simulink model "BT_da_train_cach2"  (R2017b)
(part 3 of 4)

  "IW{1,1}(98,:)'"/1 -> dotprod98/1
  dotprod98/1 -> Mux/98
  "IW{1,1}(99,:)'"/1 -> dotprod99/1
  dotprod99/1 -> Mux/99
  "IW{1,1}(100,:)'"/1 -> dotprod100/1
  dotprod100/1 -> Mux/100
  "IW{1,1}(101,:)'"/1 -> dotprod101/1
  dotprod101/1 -> Mux/101
  "IW{1,1}(102,:)'"/1 -> dotprod102/1
  dotprod102/1 -> Mux/102
  "IW{1,1}(103,:)'"/1 -> dotprod103/1
  dotprod103/1 -> Mux/103
  "IW{1,1}(104,:)'"/1 -> dotprod104/1
  dotprod104/1 -> Mux/104
  "IW{1,1}(105,:)'"/1 -> dotprod105/1
  dotprod105/1 -> Mux/105
  "IW{1,1}(106,:)'"/1 -> dotprod106/1
  dotprod106/1 -> Mux/106
  "IW{1,1}(107,:)'"/1 -> dotprod107/1
  dotprod107/1 -> Mux/107
  "IW{1,1}(108,:)'"/1 -> dotprod108/1
  dotprod108/1 -> Mux/108
  "IW{1,1}(109,:)'"/1 -> dotprod109/1
  dotprod109/1 -> Mux/109
  "IW{1,1}(110,:)'"/1 -> dotprod110/1
  dotprod110/1 -> Mux/110
  "IW{1,1}(111,:)'"/1 -> dotprod111/1
  dotprod111/1 -> Mux/111
  "IW{1,1}(112,:)'"/1 -> dotprod112/1
  dotprod112/1 -> Mux/112
  "IW{1,1}(113,:)'"/1 -> dotprod113/1
  dotprod113/1 -> Mux/113
  "IW{1,1}(114,:)'"/1 -> dotprod114/1
  dotprod114/1 -> Mux/114
  "IW{1,1}(115,:)'"/1 -> dotprod115/1
  dotprod115/1 -> Mux/115
  "IW{1,1}(116,:)'"/1 -> dotprod116/1
  dotprod116/1 -> Mux/116
  "IW{1,1}(117,:)'"/1 -> dotprod117/1
  dotprod117/1 -> Mux/117
  "IW{1,1}(118,:)'"/1 -> dotprod118/1
  dotprod118/1 -> Mux/118
  "IW{1,1}(119,:)'"/1 -> dotprod119/1
  dotprod119/1 -> Mux/119
  "IW{1,1}(120,:)'"/1 -> dotprod120/1
  dotprod120/1 -> Mux/120
  "IW{1,1}(121,:)'"/1 -> dotprod121/1
  dotprod121/1 -> Mux/121
  "IW{1,1}(122,:)'"/1 -> dotprod122/1
  dotprod122/1 -> Mux/122
  "IW{1,1}(123,:)'"/1 -> dotprod123/1
  dotprod123/1 -> Mux/123
  "IW{1,1}(124,:)'"/1 -> dotprod124/1
  dotprod124/1 -> Mux/124
  "IW{1,1}(125,:)'"/1 -> dotprod125/1
  dotprod125/1 -> Mux/125
  "IW{1,1}(126,:)'"/1 -> dotprod126/1
  dotprod126/1 -> Mux/126
  "IW{1,1}(127,:)'"/1 -> dotprod127/1
  dotprod127/1 -> Mux/127
  "IW{1,1}(128,:)'"/1 -> dotprod128/1
  dotprod128/1 -> Mux/128
  "IW{1,1}(129,:)'"/1 -> dotprod129/1
  dotprod129/1 -> Mux/129
  "IW{1,1}(130,:)'"/1 -> dotprod130/1
  dotprod130/1 -> Mux/130
  "IW{1,1}(131,:)'"/1 -> dotprod131/1
  dotprod131/1 -> Mux/131
  "IW{1,1}(132,:)'"/1 -> dotprod132/1
  dotprod132/1 -> Mux/132
  "IW{1,1}(133,:)'"/1 -> dotprod133/1
  dotprod133/1 -> Mux/133
  "IW{1,1}(134,:)'"/1 -> dotprod134/1
  dotprod134/1 -> Mux/134
  "IW{1,1}(135,:)'"/1 -> dotprod135/1
  dotprod135/1 -> Mux/135
  "IW{1,1}(136,:)'"/1 -> dotprod136/1
  dotprod136/1 -> Mux/136
  "IW{1,1}(137,:)'"/1 -> dotprod137/1
  dotprod137/1 -> Mux/137
  "IW{1,1}(138,:)'"/1 -> dotprod138/1
  dotprod138/1 -> Mux/138
  "IW{1,1}(139,:)'"/1 -> dotprod139/1
  dotprod139/1 -> Mux/139
  "IW{1,1}(140,:)'"/1 -> dotprod140/1
  dotprod140/1 -> Mux/140
  "IW{1,1}(141,:)'"/1 -> dotprod141/1
  dotprod141/1 -> Mux/141
  "IW{1,1}(142,:)'"/1 -> dotprod142/1
  dotprod142/1 -> Mux/142
  "IW{1,1}(143,:)'"/1 -> dotprod143/1
  dotprod143/1 -> Mux/143
  "IW{1,1}(144,:)'"/1 -> dotprod144/1
  dotprod144/1 -> Mux/144
  "IW{1,1}(145,:)'"/1 -> dotprod145/1
  dotprod145/1 -> Mux/145
  "IW{1,1}(146,:)'"/1 -> dotprod146/1
  dotprod146/1 -> Mux/146
  "IW{1,1}(147,:)'"/1 -> dotprod147/1
  dotprod147/1 -> Mux/147
  "IW{1,1}(148,:)'"/1 -> dotprod148/1
  dotprod148/1 -> Mux/148
  "IW{1,1}(149,:)'"/1 -> dotprod149/1
  dotprod149/1 -> Mux/149
  "IW{1,1}(150,:)'"/1 -> dotprod150/1
  dotprod150/1 -> Mux/150
  "IW{1,1}(151,:)'"/1 -> dotprod151/1
  dotprod151/1 -> Mux/151
  "IW{1,1}(152,:)'"/1 -> dotprod152/1
  dotprod152/1 -> Mux/152
  "IW{1,1}(153,:)'"/1 -> dotprod153/1
  dotprod153/1 -> Mux/153
  "IW{1,1}(154,:)'"/1 -> dotprod154/1
  dotprod154/1 -> Mux/154
  "IW{1,1}(155,:)'"/1 -> dotprod155/1
  dotprod155/1 -> Mux/155
  "IW{1,1}(156,:)'"/1 -> dotprod156/1
  dotprod156/1 -> Mux/156
  "IW{1,1}(157,:)'"/1 -> dotprod157/1
  dotprod157/1 -> Mux/157
  "IW{1,1}(158,:)'"/1 -> dotprod158/1
  dotprod158/1 -> Mux/158
  "IW{1,1}(159,:)'"/1 -> dotprod159/1
  dotprod159/1 -> Mux/159
  "IW{1,1}(160,:)'"/1 -> dotprod160/1
  dotprod160/1 -> Mux/160
  "IW{1,1}(161,:)'"/1 -> dotprod161/1
  dotprod161/1 -> Mux/161
  "IW{1,1}(162,:)'"/1 -> dotprod162/1
  dotprod162/1 -> Mux/162
  "IW{1,1}(163,:)'"/1 -> dotprod163/1
  dotprod163/1 -> Mux/163
  "IW{1,1}(164,:)'"/1 -> dotprod164/1
  dotprod164/1 -> Mux/164
  "IW{1,1}(165,:)'"/1 -> dotprod165/1
  dotprod165/1 -> Mux/165
  "IW{1,1}(166,:)'"/1 -> dotprod166/1
  dotprod166/1 -> Mux/166
  "IW{1,1}(167,:)'"/1 -> dotprod167/1
  dotprod167/1 -> Mux/167
  "IW{1,1}(168,:)'"/1 -> dotprod168/1
  dotprod168/1 -> Mux/168
  "IW{1,1}(169,:)'"/1 -> dotprod169/1
  dotprod169/1 -> Mux/169
  "IW{1,1}(170,:)'"/1 -> dotprod170/1
  dotprod170/1 -> Mux/170
  "IW{1,1}(171,:)'"/1 -> dotprod171/1
  dotprod171/1 -> Mux/171
  "IW{1,1}(172,:)'"/1 -> dotprod172/1
  dotprod172/1 -> Mux/172
  "IW{1,1}(173,:)'"/1 -> dotprod173/1
  dotprod173/1 -> Mux/173
  "IW{1,1}(174,:)'"/1 -> dotprod174/1
  dotprod174/1 -> Mux/174
  "IW{1,1}(175,:)'"/1 -> dotprod175/1
  dotprod175/1 -> Mux/175
  "IW{1,1}(176,:)'"/1 -> dotprod176/1
  dotprod176/1 -> Mux/176
  "IW{1,1}(177,:)'"/1 -> dotprod177/1
  dotprod177/1 -> Mux/177
  "IW{1,1}(178,:)'"/1 -> dotprod178/1
  dotprod178/1 -> Mux/178
  "IW{1,1}(179,:)'"/1 -> dotprod179/1
  dotprod179/1 -> Mux/179
  "IW{1,1}(180,:)'"/1 -> dotprod180/1
  dotprod180/1 -> Mux/180
  "IW{1,1}(181,:)'"/1 -> dotprod181/1
  dotprod181/1 -> Mux/181
  "IW{1,1}(182,:)'"/1 -> dotprod182/1
  dotprod182/1 -> Mux/182
  "IW{1,1}(183,:)'"/1 -> dotprod183/1
  dotprod183/1 -> Mux/183
  "IW{1,1}(184,:)'"/1 -> dotprod184/1
  dotprod184/1 -> Mux/184
  "IW{1,1}(185,:)'"/1 -> dotprod185/1
  dotprod185/1 -> Mux/185
  "IW{1,1}(186,:)'"/1 -> dotprod186/1
  dotprod186/1 -> Mux/186
  "IW{1,1}(187,:)'"/1 -> dotprod187/1
  dotprod187/1 -> Mux/187
  "IW{1,1}(188,:)'"/1 -> dotprod188/1
  dotprod188/1 -> Mux/188
  "IW{1,1}(189,:)'"/1 -> dotprod189/1
  dotprod189/1 -> Mux/189
  "IW{1,1}(190,:)'"/1 -> dotprod190/1
  dotprod190/1 -> Mux/190
  "IW{1,1}(191,:)'"/1 -> dotprod191/1
  dotprod191/1 -> Mux/191
  "IW{1,1}(192,:)'"/1 -> dotprod192/1
  dotprod192/1 -> Mux/192
  "IW{1,1}(193,:)'"/1 -> dotprod193/1
  dotprod193/1 -> Mux/193
  "IW{1,1}(194,:)'"/1 -> dotprod194/1
  dotprod194/1 -> Mux/194
  "IW{1,1}(195,:)'"/1 -> dotprod195/1
  dotprod195/1 -> Mux/195
  "IW{1,1}(196,:)'"/1 -> dotprod196/1
  dotprod196/1 -> Mux/196
  "IW{1,1}(197,:)'"/1 -> dotprod197/1
  dotprod197/1 -> Mux/197
  "IW{1,1}(198,:)'"/1 -> dotprod198/1
  dotprod198/1 -> Mux/198
  "IW{1,1}(199,:)'"/1 -> dotprod199/1
  dotprod199/1 -> Mux/199
  "IW{1,1}(200,:)'"/1 -> dotprod200/1
  dotprod200/1 -> Mux/200
  "IW{1,1}(201,:)'"/1 -> dotprod201/1
  dotprod201/1 -> Mux/201
  "IW{1,1}(202,:)'"/1 -> dotprod202/1
  dotprod202/1 -> Mux/202
  "IW{1,1}(203,:)'"/1 -> dotprod203/1
  dotprod203/1 -> Mux/203
  "IW{1,1}(204,:)'"/1 -> dotprod204/1
  dotprod204/1 -> Mux/204
  "IW{1,1}(205,:)'"/1 -> dotprod205/1
  dotprod205/1 -> Mux/205
  "IW{1,1}(206,:)'"/1 -> dotprod206/1
  dotprod206/1 -> Mux/206
  "IW{1,1}(207,:)'"/1 -> dotprod207/1
  dotprod207/1 -> Mux/207
  "IW{1,1}(208,:)'"/1 -> dotprod208/1
  dotprod208/1 -> Mux/208
  "IW{1,1}(209,:)'"/1 -> dotprod209/1
  dotprod209/1 -> Mux/209
  "IW{1,1}(210,:)'"/1 -> dotprod210/1
  dotprod210/1 -> Mux/210
  "IW{1,1}(211,:)'"/1 -> dotprod211/1
  dotprod211/1 -> Mux/211
  "IW{1,1}(212,:)'"/1 -> dotprod212/1
  dotprod212/1 -> Mux/212
  "IW{1,1}(213,:)'"/1 -> dotprod213/1
  dotprod213/1 -> Mux/213
  "IW{1,1}(214,:)'"/1 -> dotprod214/1
  dotprod214/1 -> Mux/214
  "IW{1,1}(215,:)'"/1 -> dotprod215/1
  dotprod215/1 -> Mux/215
  "IW{1,1}(216,:)'"/1 -> dotprod216/1
  dotprod216/1 -> Mux/216
  "IW{1,1}(217,:)'"/1 -> dotprod217/1
  dotprod217/1 -> Mux/217
  "IW{1,1}(218,:)'"/1 -> dotprod218/1
  dotprod218/1 -> Mux/218
  "IW{1,1}(219,:)'"/1 -> dotprod219/1
  dotprod219/1 -> Mux/219
  "IW{1,1}(220,:)'"/1 -> dotprod220/1
  dotprod220/1 -> Mux/220
  "IW{1,1}(221,:)'"/1 -> dotprod221/1
  dotprod221/1 -> Mux/221
  "IW{1,1}(222,:)'"/1 -> dotprod222/1
  dotprod222/1 -> Mux/222
  "IW{1,1}(223,:)'"/1 -> dotprod223/1
  dotprod223/1 -> Mux/223
  "IW{1,1}(224,:)'"/1 -> dotprod224/1
  dotprod224/1 -> Mux/224
  "IW{1,1}(225,:)'"/1 -> dotprod225/1
  dotprod225/1 -> Mux/225
  "IW{1,1}(226,:)'"/1 -> dotprod226/1
  dotprod226/1 -> Mux/226
  "IW{1,1}(227,:)'"/1 -> dotprod227/1
  dotprod227/1 -> Mux/227
  "IW{1,1}(228,:)'"/1 -> dotprod228/1
  dotprod228/1 -> Mux/228
  "IW{1,1}(229,:)'"/1 -> dotprod229/1
  dotprod229/1 -> Mux/229
  "IW{1,1}(230,:)'"/1 -> dotprod230/1
  dotprod230/1 -> Mux/230
  "IW{1,1}(231,:)'"/1 -> dotprod231/1
  dotprod231/1 -> Mux/231
  "IW{1,1}(232,:)'"/1 -> dotprod232/1
  dotprod232/1 -> Mux/232
  "IW{1,1}(233,:)'"/1 -> dotprod233/1
  dotprod233/1 -> Mux/233
  "IW{1,1}(234,:)'"/1 -> dotprod234/1
  dotprod234/1 -> Mux/234
  "IW{1,1}(235,:)'"/1 -> dotprod235/1
  dotprod235/1 -> Mux/235
  "IW{1,1}(236,:)'"/1 -> dotprod236/1
  dotprod236/1 -> Mux/236
  "IW{1,1}(237,:)'"/1 -> dotprod237/1
  dotprod237/1 -> Mux/237
  "IW{1,1}(238,:)'"/1 -> dotprod238/1
  dotprod238/1 -> Mux/238
  "IW{1,1}(239,:)'"/1 -> dotprod239/1
  dotprod239/1 -> Mux/239
  "IW{1,1}(240,:)'"/1 -> dotprod240/1
  dotprod240/1 -> Mux/240
  "IW{1,1}(241,:)'"/1 -> dotprod241/1
  dotprod241/1 -> Mux/241
  "IW{1,1}(242,:)'"/1 -> dotprod242/1
  dotprod242/1 -> Mux/242
  "IW{1,1}(243,:)'"/1 -> dotprod243/1
  dotprod243/1 -> Mux/243
  "IW{1,1}(244,:)'"/1 -> dotprod244/1
  dotprod244/1 -> Mux/244
  "IW{1,1}(245,:)'"/1 -> dotprod245/1
  dotprod245/1 -> Mux/245
  "IW{1,1}(246,:)'"/1 -> dotprod246/1
  dotprod246/1 -> Mux/246
  "IW{1,1}(247,:)'"/1 -> dotprod247/1
  dotprod247/1 -> Mux/247
  "IW{1,1}(248,:)'"/1 -> dotprod248/1
  dotprod248/1 -> Mux/248
  "IW{1,1}(249,:)'"/1 -> dotprod249/1
  dotprod249/1 -> Mux/249
  "IW{1,1}(250,:)'"/1 -> dotprod250/1
  dotprod250/1 -> Mux/250
  "IW{1,1}(251,:)'"/1 -> dotprod251/1
  dotprod251/1 -> Mux/251
  "IW{1,1}(252,:)'"/1 -> dotprod252/1
  dotprod252/1 -> Mux/252
  "IW{1,1}(253,:)'"/1 -> dotprod253/1
  dotprod253/1 -> Mux/253
  "IW{1,1}(254,:)'"/1 -> dotprod254/1
  dotprod254/1 -> Mux/254
  "IW{1,1}(255,:)'"/1 -> dotprod255/1
  dotprod255/1 -> Mux/255
  "IW{1,1}(256,:)'"/1 -> dotprod256/1
  dotprod256/1 -> Mux/256
  "IW{1,1}(257,:)'"/1 -> dotprod257/1
  dotprod257/1 -> Mux/257
  "IW{1,1}(258,:)'"/1 -> dotprod258/1
  dotprod258/1 -> Mux/258
  "IW{1,1}(259,:)'"/1 -> dotprod259/1
  dotprod259/1 -> Mux/259
  "IW{1,1}(260,:)'"/1 -> dotprod260/1
  dotprod260/1 -> Mux/260
  "IW{1,1}(261,:)'"/1 -> dotprod261/1
  dotprod261/1 -> Mux/261
  "IW{1,1}(262,:)'"/1 -> dotprod262/1
  dotprod262/1 -> Mux/262
  "IW{1,1}(263,:)'"/1 -> dotprod263/1
  dotprod263/1 -> Mux/263
  "IW{1,1}(264,:)'"/1 -> dotprod264/1
  dotprod264/1 -> Mux/264
  "IW{1,1}(265,:)'"/1 -> dotprod265/1
  dotprod265/1 -> Mux/265
  "IW{1,1}(266,:)'"/1 -> dotprod266/1
  dotprod266/1 -> Mux/266
  "IW{1,1}(267,:)'"/1 -> dotprod267/1
  dotprod267/1 -> Mux/267
  "IW{1,1}(268,:)'"/1 -> dotprod268/1
  dotprod268/1 -> Mux/268
  "IW{1,1}(269,:)'"/1 -> dotprod269/1
  dotprod269/1 -> Mux/269
  "IW{1,1}(270,:)'"/1 -> dotprod270/1
  dotprod270/1 -> Mux/270
  "IW{1,1}(271,:)'"/1 -> dotprod271/1
  dotprod271/1 -> Mux/271
  "IW{1,1}(272,:)'"/1 -> dotprod272/1
  dotprod272/1 -> Mux/272
  "IW{1,1}(273,:)'"/1 -> dotprod273/1
  dotprod273/1 -> Mux/273
  "IW{1,1}(274,:)'"/1 -> dotprod274/1
  dotprod274/1 -> Mux/274
  "IW{1,1}(275,:)'"/1 -> dotprod275/1
  dotprod275/1 -> Mux/275
  "IW{1,1}(276,:)'"/1 -> dotprod276/1
  dotprod276/1 -> Mux/276
  "IW{1,1}(277,:)'"/1 -> dotprod277/1
  dotprod277/1 -> Mux/277
  "IW{1,1}(278,:)'"/1 -> dotprod278/1
  dotprod278/1 -> Mux/278
  "IW{1,1}(279,:)'"/1 -> dotprod279/1
  dotprod279/1 -> Mux/279
  "IW{1,1}(280,:)'"/1 -> dotprod280/1
  dotprod280/1 -> Mux/280
  "IW{1,1}(281,:)'"/1 -> dotprod281/1
  dotprod281/1 -> Mux/281
  "IW{1,1}(282,:)'"/1 -> dotprod282/1
  dotprod282/1 -> Mux/282
  "IW{1,1}(283,:)'"/1 -> dotprod283/1
  dotprod283/1 -> Mux/283
  "IW{1,1}(284,:)'"/1 -> dotprod284/1
  dotprod284/1 -> Mux/284
  "IW{1,1}(285,:)'"/1 -> dotprod285/1
  dotprod285/1 -> Mux/285
  "IW{1,1}(286,:)'"/1 -> dotprod286/1
  dotprod286/1 -> Mux/286
  "IW{1,1}(287,:)'"/1 -> dotprod287/1
  dotprod287/1 -> Mux/287
  "IW{1,1}(288,:)'"/1 -> dotprod288/1
  dotprod288/1 -> Mux/288
  "IW{1,1}(289,:)'"/1 -> dotprod289/1
  dotprod289/1 -> Mux/289
  "IW{1,1}(290,:)'"/1 -> dotprod290/1
  dotprod290/1 -> Mux/290
  "IW{1,1}(291,:)'"/1 -> dotprod291/1
  dotprod291/1 -> Mux/291
  "IW{1,1}(292,:)'"/1 -> dotprod292/1
  dotprod292/1 -> Mux/292
  "IW{1,1}(293,:)'"/1 -> dotprod293/1
  dotprod293/1 -> Mux/293
  "IW{1,1}(294,:)'"/1 -> dotprod294/1
  dotprod294/1 -> Mux/294
  "IW{1,1}(295,:)'"/1 -> dotprod295/1
  dotprod295/1 -> Mux/295
  "IW{1,1}(296,:)'"/1 -> dotprod296/1
  dotprod296/1 -> Mux/296
  "IW{1,1}(297,:)'"/1 -> dotprod297/1
  dotprod297/1 -> Mux/297
  "IW{1,1}(298,:)'"/1 -> dotprod298/1
  dotprod298/1 -> Mux/298
  "IW{1,1}(299,:)'"/1 -> dotprod299/1
  dotprod299/1 -> Mux/299
  "IW{1,1}(300,:)'"/1 -> dotprod300/1
  dotprod300/1 -> Mux/300
  Mux/1 -> "iz{1,1}"/1
